simulink model "pmsm_model"  (R2022b)
settings: Solver=VariableStepAuto  StartTime=0.0  StopTime=10  RelTol=1e-3
values from neighbouring files (symbols this model uses):
  controller_gain = K(:,:,1)    [Simulink_Tsiamis.m]    (also in Simulink_leqg.m = L(:,:,1)*B'*P_tilde(:,:,1)*A; Simulink_lqr.m = L(:,:,1)*B'*P(:,:,1)*A)
  controller_offset = l(:,1) + h(:,1)    [Simulink_Tsiamis.m]    (also in Simulink_leqg.m = L(:,:,1)*B'*(P_tilde(:,:,1)*D*tl_mean + K(:,:,1)*s(:,1)); Simulink_lqr.m = L(:,:,1)*B'*s(:,1))
  idss = 0    [LEQG_Gaussian.m]    (also in LEQG_simulink_find_theta.m; LEQG_single_run.m; LQR_Gaussian.m; LQR_single_run.m)
  iqss = 2*(Br*omegass + tl_mean)/(3*psi_ro)    (= 1.2888574359)    [LEQG_Gaussian.m]    (also in LEQG_simulink_find_theta.m = 0.507332429575; LEQG_single_run.m; LQR_Gaussian.m; LQR_single_run.m)
  omegass = omega_sync    (= 314.159)    [LEQG_Gaussian.m]    (also in LEQG_simulink_find_theta.m = 157.079632679; LEQG_single_run.m; LQR_Gaussian.m; LQR_single_run.m)
  p = 5    [LEQG_simulink_find_theta.m]    (also in Simulink_Tsiamis.m; Simulink_leqg.m; Simulink_lqr.m; Tsiamis_simulink_find_mu.m)
  tl_mean = 0    [LEQG_Gaussian.m]    (also in LEQG_simulink_find_theta.m; LEQG_single_run.m; LQR_Gaussian.m; LQR_single_run.m)
  tl_sd = 2    [LEQG_Gaussian.m]    (also in LEQG_simulink_find_theta.m = 1; LEQG_single_run.m; LQR_Gaussian.m; LQR_single_run.m = 1)
  vdss = - Lq * omegass * iqss    (= -0.323924930563)    [LEQG_Gaussian.m]    (also in LEQG_simulink_find_theta.m = -0.577764039709; LEQG_single_run.m; LQR_Gaussian.m; LQR_single_run.m)
  vqss = omegass * psi_ro + Rs * iqss    (= 204.261348585)    [LEQG_Gaussian.m]    (also in LEQG_simulink_find_theta.m = 129.72577533; LEQG_single_run.m; LQR_Gaussian.m; LQR_single_run.m)
libraries: nesl_utility x7, fl_lib x6, ee_lib x3, eeTransforms x2
settings Model: Creator=wangy  LastModifiedBy=wangy

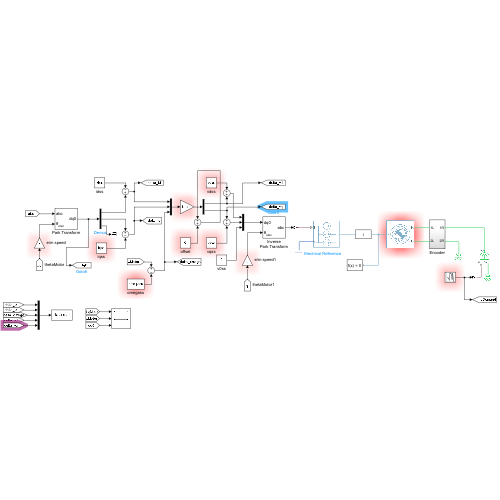
[thumbnail: Simulink's stored preview of the top-level diagram]
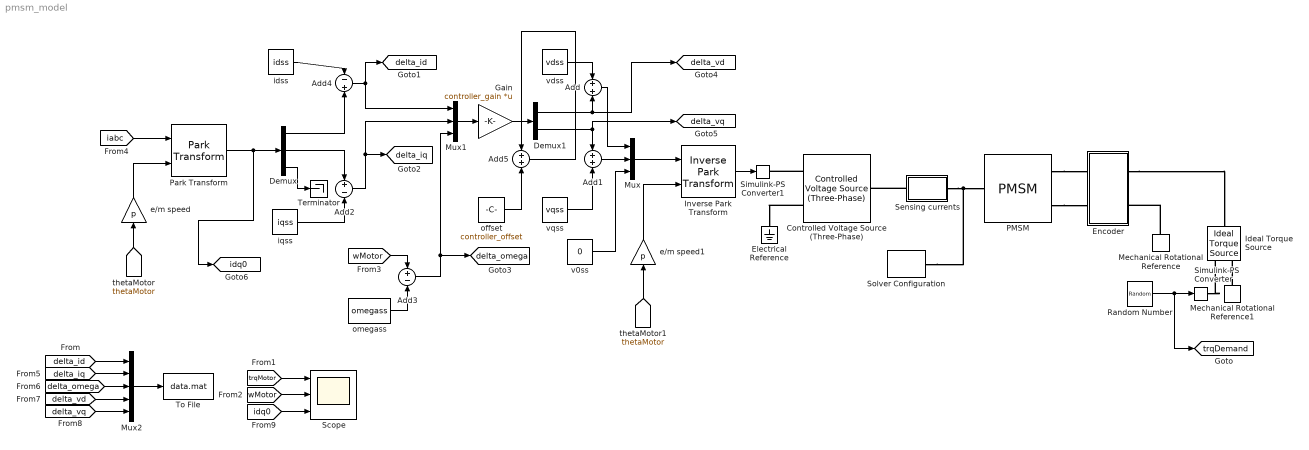
== system pmsm_model ==
  Add : Sum
  Add1 : Sum
  Add2 : Sum  Inputs=+-
  Add3 : Sum  Inputs=+-
  Add4 : Sum  Inputs=-+
  Add5 : Sum
  Controlled Voltage Source (Three-Phase) : ee_lib/Sources/Controlled Voltage Source (Three-Phase)  input_option=ee.enum.inputType.instantaneous  FRated=60 Hz
      settings: InternalSimscapePortConfiguration="{\"Bottom\":[],\"Left\":[{\"id\":\"S\",\"label\":\"S\",\"type\":\"input\"},{\"id\":\"n\",\"label\":\"n\",\"type\":\"foundation.electrical.electrical\"}],\"Right\":[{\"id\":\"N\",\"label\":\"~\",\"type\":\"foundation.electrical.three_phase\"}],\"Top\":[]}"
  Demux : Demux  Outputs=3
  Demux1 : Demux  Outputs=2
  Electrical Reference : fl_lib/Electrical/Electrical Elements/Electrical Reference
  Encoder : Subsystem
  Gain : Gain  Gain=controller_gain  Multiplication=Matrix(K*u)
  Ideal Torque Source : fl_lib/Mechanical/Mechanical Sources/Ideal Torque Source
  Inverse Park Transform : eeTransforms/Inverse Park Transform  AxisAlignment=D-axis  PowerInvariant=off
      settings: LibrarySourceBlock=|
      | ee_sl_lib/Mathematical
      | Transforms/Inverse
      | Park Transform
  Mechanical Rotational Reference : fl_lib/Mechanical/Rotational Elements/Mechanical Rotational Reference
  Mechanical Rotational Reference1 : fl_lib/Mechanical/Rotational Elements/Mechanical Rotational Reference
  Mux : Mux  Inputs=3
  Mux1 : Mux  Inputs=3
  Mux2 : Mux  Inputs=5
  PMSM : ee_lib/Electromechanical/Permanent Magnet/PMSM  port_option=ee.enum.threePhasePort.composite  winding_type=ee.enum.statorconnection.wye  machine_param=ee.enum.pmsm.parameterization.constant  nPolePairs=5  pmflux_param=ee.enum.pmflux.fluxlinkage  pm_flux_linkage=0.165139782501293 Wb  torque_constant=0.825698912506463 N*m/A  back_emf_constant=0.825698912506463 V/(rad/s)  stator_param=ee.enum.statorparam.LdLqL0  Ld=0.00145 H  Lq=0.00145 H  idVec=[-200 0 200] % Parameter not set A  iqVec=[-200 0 200] % Parameter not set A  LdMatrix=[0.0002 0.0002 0.0002;0.0002 0.0002 0.0002;0.0002 0.0002 0.0002] % Parameter not set H  LqMatrix=[0.0002 0.0002 0.0002;0.0002 0.0002 0.0002;0.0002 0.0002 0.0002] % Parameter not set H  PmMatrix=[0.1 0.1 0.1;0.1 0.1 0.1;0.1 0.1 0.1] Wb  ktMatrix=[0.18 0.18 0.18;0.18 0.18 0.18;0.18 0.18 0.18] N*m/A  keMatrix=[0.18 0.18 0.18;0.18 0.18 0.18;0.18 0.18 0.18] % Parameter not set V/(rad/s)  L0=[] % Parameter not set H  Ls=0.0002 H  Lm=-2e-05 H  Ms=2e-05 H  Rs=0.065 Ohm  zero_sequence=ee.enum.park.zerosequence.exclude  axes_param=ee.enum.rotorangle.daxis  loss_param=ee.enum.ironloss.none  losses_oc=[0 0 0] % Parameter not set W  losses_sc=[0 0 0] % Parameter not set W  f_losses=60 % Parameter not set Hz  Isc_losses=95 % Parameter not set A  J=0.00821 kg*m^2  lam=0.004 N*m/(rad/s)  i_d_specify=on  i_d_priority=High  i_d=idss A  i_d_nominal_specify=off  i_d_nominal_unit=A  i_d_nominal_value=1  i_q_specify=on  i_q_priority=High  i_q=iqss A  i_q_nominal_specify=off  i_q_nominal_unit=A  i_q_nominal_value=1  torque_specify=on  torque_priority=Low  torque=tl_mean N*m  torque_nominal_specify=off  torque_nominal_unit=N*m  torque_nominal_value=1  angular_velocity_specify=on  angular_velocity_priority=High  angular_velocity=omega_rpm rpm  angular_velocity_nominal_specify=off  angular_velocity_nominal_unit=rpm  angular_velocity_nominal_value=1  angular_position_specify=off  angular_position_priority=High  angular_position=0 deg  angular_position_nominal_specify=off  angular_position_nominal_unit=deg  angular_position_nominal_value=1  alpha=3.93e-3 1/K  alpha_flux=-0.001 1/K  Tmeas=298.15 K  stator_thermal_mass=100 J/K  rotor_thermal_mass=200 J/K  Rm_percent_rotor=90  Rd_percent_rotor=30  temperatureA_specify=off  temperatureA_priority=High  temperatureA=25 degC  temperatureA_nominal_specify=off  temperatureA_nominal_unit=degC  temperatureA_nominal_value=1  temperatureB_specify=off  temperatureB_priority=High  temperatureB=25 degC  temperatureB_nominal_specify=off  temperatureB_nominal_unit=degC  temperatureB_nominal_value=1  temperatureC_specify=off  temperatureC_priority=High  temperatureC=25 degC  temperatureC_nominal_specify=off  temperatureC_nominal_unit=degC  temperatureC_nominal_value=1  temperatureR_specify=off  temperatureR_priority=High  temperatureR=25 degC  temperatureR_nominal_specify=off  temperatureR_nominal_unit=degC  temperatureR_nominal_value=1
      settings: InternalSimscapePortConfiguration="{\"Bottom\":[],\"Left\":[{\"id\":\"N\",\"label\":\"~\",\"type\":\"foundation.electrical.three_phase\"}],\"Right\":[{\"id\":\"R\",\"label\":\"R\",\"type\":\"foundation.mechanical.rotational.rotational\"},{\"id\":\"C\",\"label\":\"C\",\"type\":\"foundation.mechanical.rotational.rotational\"}],\"Top\":[]}"
  Park Transform : eeTransforms/Park Transform  AxisAlignment=D-axis  PowerInvariant=off
      settings: LibrarySourceBlock=|
      | ee_sl_lib/Mathematical
      | Transforms/Park Transform
  Random Number : RandomNumber  Mean=tl_mean  Variance=tl_sd^2  SampleTime=1e-3
  Scope : Scope  NumInputPorts=3
  Sensing currents : Subsystem
      mask Display: disp('i')
  Simulink-PS Converter : nesl_utility/Simulink-PS Converter  PhysicalDomain=network_engine_domain  SubClassName=ps_input  LeftPortType=input  RightPortType=output  PseudoPeriodic=off  Frequencies=[]  NoiseDistribution=none  NoiseParameters=[]  Unit=1  AffineConversion=off  FilteringAndDerivatives=provide  SimscapeFilterOrder=1  InputFilterTimeConstant=0.001  UdotUserProvided=0
  Simulink-PS Converter1 : nesl_utility/Simulink-PS Converter  PhysicalDomain=network_engine_domain  SubClassName=ps_input  LeftPortType=input  RightPortType=output  PseudoPeriodic=off  Frequencies=[]  NoiseDistribution=none  NoiseParameters=[]  Unit=1  AffineConversion=off  FilteringAndDerivatives=provide  SimscapeFilterOrder=1  InputFilterTimeConstant=0.001  UdotUserProvided=0
  Solver Configuration : nesl_utility/Solver Configuration  PhysicalDomain=network_engine_domain  SubClassName=solver  LeftPortType=input  RightPortType=generic  Tones=[]  Harmonics=[]  SimulateNoise=off  Profile=off  UseLocalSampling=off  EnableSwitchedLinearOptims=on  FrequencyDomain=off  UseCCode=off  RelTol=0.001  AbsTol=0.001  MinStep=1e-09  ToWorkspace=off  RevertToSquareIcSolve=off  NumHomotopyIterations=100  PhasorMode=off  PhasorModeNumHarmonics=1  ConsistencySolver=NEWTON_XTOL_AFTER_FTOL  IndexReductionMethod=DerivativeReplacement  DoDC=off  ResidualTolerance=1e-09  ConsistencyTolSource=GLOBAL  ConsistencyAbsTol=0.001  ConsistencyRelTol=0.001  ConsistencyTolFactor=0.001  UseLocalSolver=off  LocalSolverChoice=NE_BACKWARD_EULER_ADVANCER  ResolveIndetEquations=on  FunctionEvalNumThread=1  LocalSolverSampleTime=0.001  DoFixedCost=off  MaxNonlinIter=3  MaxModeIter=2  ComputeImpulses=off  ImpulseIterations=2  LinearAlgebra=auto  LinearAlgebraNumThread=0  EquationFormulation=NE_TIME_EF  DelaysMemoryBudget=1024  AutomaticFiltering=on  FilteringTimeConstant=0.001  PartitionStorageMethod=AS_NEEDED  PartitionMemoryBudget=1024  PartitionMethod=ROBUST
  Terminator : Terminator
  To File : ToFile  Filename=data.mat
  e/m speed : Gain  Gain=p
  e/m speed1 : Gain  Gain=p
  idss : Constant  Value=idss
  iqss : Constant  Value=iqss
  offset : Constant  Value=controller_offset
  omegass : Constant  Value=omegass
  v0ss : Constant  Value=0
  vdss : Constant  Value=vdss
  vqss : Constant  Value=vqss
  tag scope: delta_id=global, delta_iq=global, delta_omega=global, delta_vd=global, delta_vq=global, idq0=global, trqDemand=global
  wires:
  Random Number/1 -> [trqDemand], Simulink-PS Converter/1
  Inverse Park Transform/1 -> Simulink-PS Converter1/1
  Mux/1 -> Inverse Park Transform/1
  v0ss/1 -> Mux/3
  [trqMotor] -> Scope/1
  [wMotor] -> Scope/2
  [iabc] -> Park Transform/1
  e/m speed/1 -> Park Transform/2
  [thetaMotor] -> e/m speed/1
  Park Transform/1 -> [idq0], Demux/1
  [thetaMotor] -> e/m speed1/1
  e/m speed1/1 -> Inverse Park Transform/2
  Demux/3 -> Terminator/1
  Demux/1 -> Add4/2
  idss/1 -> Add4/1
  vdss/1 -> Add/1
  Add/1 -> Mux/1
  Add4/1 -> [delta_id], Mux1/1
  Mux1/1 -> Gain/1
  Demux/2 -> Add2/1
  iqss/1 -> Add2/2
  Add2/1 -> [delta_iq], Mux1/2
  [wMotor] -> Add3/1
  omegass/1 -> Add3/2
  Add3/1 -> Mux1/3, [delta_omega]
  Demux1/1 -> [delta_vd], Add/2
  Demux1/2 -> [delta_vq], Add1/1
  vqss/1 -> Add1/2
  Add1/1 -> Mux/2
  offset/1 -> Add5/2
  Gain/1 -> Add5/1
  Add5/1 -> Demux1/1
  Mux2/1 -> To File/1
  [delta_id] -> Mux2/1
  [delta_iq] -> Mux2/2
  [delta_omega] -> Mux2/3
  [delta_vd] -> Mux2/4
  [delta_vq] -> Mux2/5
  [idq0] -> Scope/3
  connections:
  Mechanical Rotational Reference/LConn1 -- Encoder/RConn2
  Sensing currents/LConn1 -- Controlled Voltage Source (Three-Phase)/RConn1
  Simulink-PS Converter/RConn1 -- Ideal Torque Source/RConn1
  Encoder/RConn1 -- Ideal Torque Source/LConn1
  Mechanical Rotational Reference1/LConn1 -- Ideal Torque Source/RConn2
  PMSM/RConn1 -- Encoder/LConn1
  Sensing currents/RConn1 -- Solver Configuration/RConn1 -- PMSM/LConn1
  PMSM/RConn2 -- Encoder/LConn2
  Controlled Voltage Source (Three-Phase)/LConn1 -- Simulink-PS Converter1/RConn1
  Controlled Voltage Source (Three-Phase)/LConn2 -- Electrical Reference/LConn1

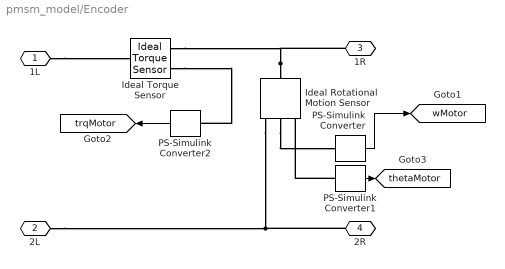
== system pmsm_model/Encoder ==
  Ideal Rotational Motion Sensor : fl_lib/Mechanical/Mechanical Sensors/Ideal Rotational Motion Sensor  reference=foundation.enum.MeasurementReference.difference  acceleration_port=false  velocity_port=true  position_port=true  wrap_angle=simscape.enum.onoff.off  offset=0 deg
  Ideal Torque Sensor : fl_lib/Mechanical/Mechanical Sensors/Ideal Torque Sensor
  PS-Simulink Converter : nesl_utility/PS-Simulink Converter  PhysicalDomain=network_engine_domain  SubClassName=ps_output  LeftPortType=input  RightPortType=output  PseudoPeriodic=off  Frequencies=[]  VectorFormat=1-D array  Unit=rad/s  AffineConversion=off
  PS-Simulink Converter1 : nesl_utility/PS-Simulink Converter  PhysicalDomain=network_engine_domain  SubClassName=ps_output  LeftPortType=input  RightPortType=output  PseudoPeriodic=off  Frequencies=[]  VectorFormat=1-D array  Unit=rad  AffineConversion=off
  PS-Simulink Converter2 : nesl_utility/PS-Simulink Converter  PhysicalDomain=network_engine_domain  SubClassName=ps_output  LeftPortType=input  RightPortType=output  PseudoPeriodic=off  Frequencies=[]  VectorFormat=1-D array  Unit=N*m  AffineConversion=off
  1L : PMIOPort  Side=Left
  2L : PMIOPort  Port=2  Side=Left
  1R : PMIOPort  Port=3  Side=Right
  2R : PMIOPort  Port=4  Side=Right
  tag scope: thetaMotor=global, trqMotor=global, wMotor=global
  wires:
  PS-Simulink Converter2/1 -> [trqMotor]
  PS-Simulink Converter/1 -> [wMotor]
  PS-Simulink Converter1/1 -> [thetaMotor]
  connections:
  Ideal Torque Sensor/RConn2 -- PS-Simulink Converter2/LConn1
  1L/RConn1 -- Ideal Torque Sensor/LConn1
  2R/RConn1 -- 2L/RConn1 -- Ideal Rotational Motion Sensor/RConn1
  Ideal Rotational Motion Sensor/LConn1 -- 1R/RConn1 -- Ideal Torque Sensor/RConn1
  Ideal Rotational Motion Sensor/RConn2 -- PS-Simulink Converter/LConn1
  PS-Simulink Converter1/LConn1 -- Ideal Rotational Motion Sensor/RConn3

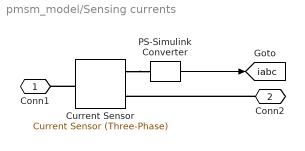
== system pmsm_model/Sensing currents ==
  Current Sensor : ee_lib/Sensors & Transducers/Current Sensor (Three-Phase)
  PS-Simulink Converter : nesl_utility/PS-Simulink Converter  PhysicalDomain=network_engine_domain  SubClassName=ps_output  LeftPortType=input  RightPortType=output  PseudoPeriodic=off  Frequencies=[]  VectorFormat=1-D array  Unit=A  AffineConversion=off
  Conn1 : PMIOPort  Side=Left
  Conn2 : PMIOPort  Port=2  Side=Right
  tag scope: iabc=global
  wires:
  PS-Simulink Converter/1 -> [iabc]
  connections:
  Current Sensor/RConn1 -- PS-Simulink Converter/LConn1
  Conn2/RConn1 -- Current Sensor/RConn2
  Current Sensor/LConn1 -- Conn1/RConn1
